simulink model "FMS"  (R2021b)
settings: Solver=VariableStepAuto  StartTime=0.0  StopTime=10.0  RelTol=1e-3
model workspace (MAT data in the model file):
  Control_State_In = Simulink.Bus
  Control_State_In.Alignment = -1
  Control_State_In.PreserveElementDimensions = 0
  Control_State_In.Elements_internal(1) = Simulink.BusElement
  Control_State_In.Elements_internal(1).DimensionsMode = 'Fixed'
  Control_State_In.Elements_internal(1).SamplingMode = 'Sample based'
  Control_State_In.Elements_internal(1).SampleTime = -1
  Control_State_In.Elements_internal(1).Description = 'position'
  Control_State_In.Elements_internal(1).Name = 'x'
  Control_State_In.Elements_internal(1).DataType_internal = 'double'
  Control_State_In.Elements_internal(1).Complexity = 'real'
  Control_State_In.Elements_internal(1).Dimensions = 1
  Control_State_In.Elements_internal(2) = Simulink.BusElement
  Control_State_In.Elements_internal(2).DimensionsMode = 'Fixed'
  Control_State_In.Elements_internal(2).SamplingMode = 'Sample based'
  Control_State_In.Elements_internal(2).SampleTime = -1
  Control_State_In.Elements_internal(2).Description = 'position'
  Control_State_In.Elements_internal(2).Name = 'y'
  Control_State_In.Elements_internal(2).DataType_internal = 'double'
  Control_State_In.Elements_internal(2).Complexity = 'real'
  Control_State_In.Elements_internal(2).Dimensions = 1
  Control_State_In.Elements_internal(3) = Simulink.BusElement
  Control_State_In.Elements_internal(3).DimensionsMode = 'Fixed'
  Control_State_In.Elements_internal(3).SamplingMode = 'Sample based'
  Control_State_In.Elements_internal(3).SampleTime = -1
  Control_State_In.Elements_internal(3).Description = 'cap'
  Control_State_In.Elements_internal(3).Name = 'fpa'
  Control_State_In.Elements_internal(3).DataType_internal = 'double'
  Control_State_In.Elements_internal(3).Complexity = 'real'
  Control_State_In.Elements_internal(3).Dimensions = 1
  Control_State_In.Elements_internal(4) = Simulink.BusElement
  Control_State_In.Elements_internal(4).DimensionsMode = 'Fixed'
  Control_State_In.Elements_internal(4).SamplingMode = 'Sample based'
  Control_State_In.Elements_internal(4).SampleTime = -1
  Control_State_In.Elements_internal(4).Description = 'altitude'
  Control_State_In.Elements_internal(4).Name = 'z'
  Control_State_In.Elements_internal(4).DataType_internal = 'double'
  Control_State_In.Elements_internal(4).Complexity = 'real'
  Control_State_In.Elements_internal(4).Dimensions = 1
  Control_State_In.Elements_internal(5) = Simulink.BusElement
  Control_State_In.Elements_internal(5).DimensionsMode = 'Fixed'
  Control_State_In.Elements_internal(5).SamplingMode = 'Sample based'
  Control_State_In.Elements_internal(5).SampleTime = -1
  Control_State_In.Elements_internal(5).Description = 'vitesse'
  Control_State_In.Elements_internal(5).Name = 'Vp'
  Control_State_In.Elements_internal(5).DataType_internal = 'double'
  Control_State_In.Elements_internal(5).Complexity = 'real'
  Control_State_In.Elements_internal(5).Dimensions = 1
  Control_State_In.Elements_internal(6) = Simulink.BusElement
  Control_State_In.Elements_internal(6).DimensionsMode = 'Fixed'
  Control_State_In.Elements_internal(6).SamplingMode = 'Sample based'
  Control_State_In.Elements_internal(6).SampleTime = -1
  Control_State_In.Elements_internal(6).Description = 'roulis'
  Control_State_In.Elements_internal(6).Name = 'phi'
  Control_State_In.Elements_internal(6).DataType_internal = 'double'
  Control_State_In.Elements_internal(6).Complexity = 'real'
  Control_State_In.Elements_internal(6).Dimensions = 1
  Control_State_In.Elements_internal(7) = Simulink.BusElement
  Control_State_In.Elements_internal(7).DimensionsMode = 'Fixed'
  Control_State_In.Elements_internal(7).SamplingMode = 'Sample based'
  Control_State_In.Elements_internal(7).SampleTime = -1
  Control_State_In.Elements_internal(7).Description = 'lacet'
  Control_State_In.Elements_internal(7).Name = 'psi'
  Control_State_In.Elements_internal(7).DataType_internal = 'double'
  Control_State_In.Elements_internal(7).Complexity = 'real'
  Control_State_In.Elements_internal(7).Dimensions = 1
  Control_State_In.DataScope = 'Auto'
  Pilot_Input = Simulink.Bus
  Pilot_Input.Alignment = -1
  Pilot_Input.PreserveElementDimensions = 0
  Pilot_Input.Elements_internal = Simulink.BusElement
  Pilot_Input.Elements_internal.DimensionsMode = 'Fixed'
  Pilot_Input.Elements_internal.SamplingMode = 'Sample based'
  Pilot_Input.Elements_internal.SampleTime = -1
  Pilot_Input.Elements_internal.Description = 'choix de mode FCU par le pilote'
  Pilot_Input.Elements_internal.Name = 'FCU_lateral_mode'
  Pilot_Input.Elements_internal.DataType_internal = 'int8'
  Pilot_Input.Elements_internal.Complexity = 'real'
  Pilot_Input.Elements_internal.Dimensions = 1
  Pilot_Input.DataScope = 'Auto'
settings Model: Creator=lhubl  LastModifiedBy=Paul

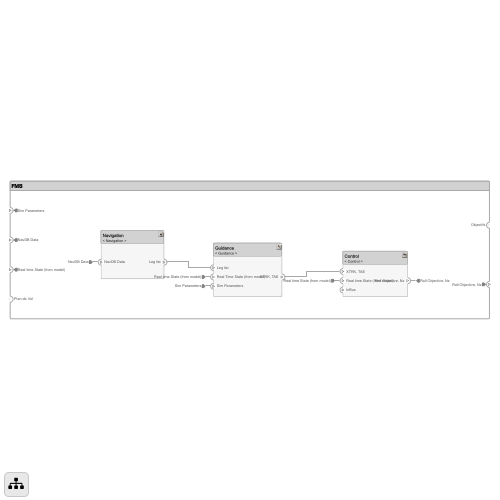
[thumbnail: Simulink's stored preview of the top-level diagram]
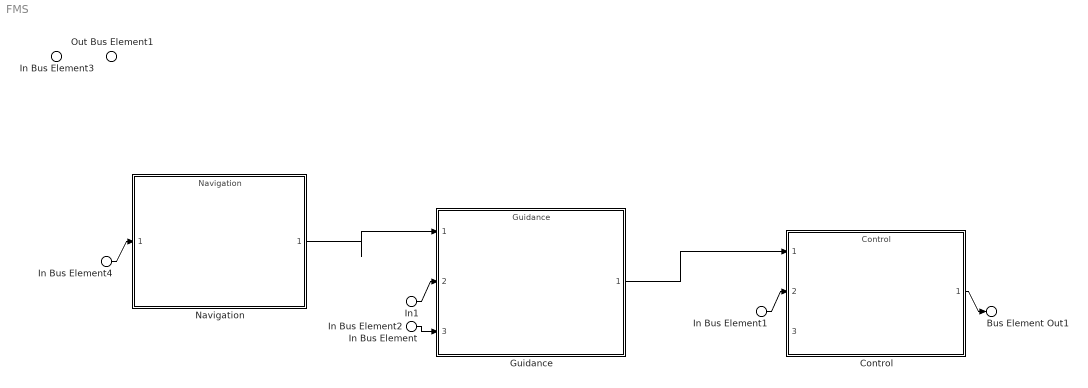
== system FMS ==
  In Bus Element : Inport  PortName=Sim Parameters
  In Bus Element4 : Inport  Port=2  PortName=NavDB Data
  In Bus Element1 : Inport  Port=3  PortName=Real time State (from model)
  In Bus Element2 : Inport  Port=3  PortName=Real time State (from model)
  In1 : Inport  Port=3  PortName=Real time State (from model)
  In Bus Element3 : Inport  Port=4  PortName=Plan de Vol
  Control : ModelReference  ModelNameDialog=Control  SimulationMode=Normal  ModelReferenceVersion=1.4
      settings: PortSchema="{\"entries\":[{\"content\":{\"headerSize\":38,\"margin\":15,\"minimumSpacing\":25,\"sides\":[{\"content\":{\"connectorIds\":[\"In1\",\"In2\",\"In3\"]},\"type\":\"ConnectorPlacement.EquallySpacedRectSide\",\"uuid\":\"f0697a98-65c4-48b6-9148-6d90a1a908b8\"},{\"content\":{\"connectorIds\":[\"Out1\"],\"side\":\"RIGHT\"},\"type\":\"ConnectorPlacement.EquallySpacedRectSide\",\"uuid\":\"c62a382e-4014-433d-b035-2a8a1906ece2\"},{\"content\":{\"connectorIds\":[],\"side\":\"TOP\"},\"type\":\"ConnectorPlacement.EquallySpacedRectSide\",\"uuid\":\"02cc979b-05b8-4cbd-9662-94fbd431603b\"}]},\"type\":\"ConnectorPlacement.EquallySpacedConnector\",\"uuid\":\"1201885f-d543-4e5c-981e-efbc8a5dca28\"}],\"packageUris\":[\"http://schema.mathworks.com/mf0/Connector/R2020b\"],\"version\":\"1.0\"}"
  "Guidance " : ModelReference  ModelNameDialog=Guidance  SimulationMode=Normal  ModelReferenceVersion=1.11
      settings: PortSchema="{\"entries\":[{\"content\":{\"headerSize\":38,\"margin\":15,\"minimumSpacing\":25,\"sides\":[{\"content\":{\"connectorIds\":[\"In1\",\"In2\",\"In3\"]},\"type\":\"ConnectorPlacement.EquallySpacedRectSide\",\"uuid\":\"f0697a98-65c4-48b6-9148-6d90a1a908b8\"},{\"content\":{\"connectorIds\":[\"Out1\"],\"side\":\"RIGHT\"},\"type\":\"ConnectorPlacement.EquallySpacedRectSide\",\"uuid\":\"c62a382e-4014-433d-b035-2a8a1906ece2\"},{\"content\":{\"connectorIds\":[],\"side\":\"TOP\"},\"type\":\"ConnectorPlacement.EquallySpacedRectSide\",\"uuid\":\"02cc979b-05b8-4cbd-9662-94fbd431603b\"}]},\"type\":\"ConnectorPlacement.EquallySpacedConnector\",\"uuid\":\"1201885f-d543-4e5c-981e-efbc8a5dca28\"}],\"packageUris\":[\"http://schema.mathworks.com/mf0/Connector/R2020b\"],\"version\":\"1.0\"}"
  Navigation : ModelReference  ModelNameDialog=Navigation  SimulationMode=Normal  ModelReferenceVersion=1.3
      settings: PortSchema="{\"entries\":[{\"content\":{\"headerSize\":38,\"margin\":15,\"minimumSpacing\":25,\"sides\":[{\"content\":{\"connectorIds\":[\"In1\"]},\"type\":\"ConnectorPlacement.EquallySpacedRectSide\",\"uuid\":\"f0697a98-65c4-48b6-9148-6d90a1a908b8\"},{\"content\":{\"connectorIds\":[\"Out1\"],\"side\":\"RIGHT\"},\"type\":\"ConnectorPlacement.EquallySpacedRectSide\",\"uuid\":\"c62a382e-4014-433d-b035-2a8a1906ece2\"},{\"content\":{\"connectorIds\":[],\"side\":\"TOP\"},\"type\":\"ConnectorPlacement.EquallySpacedRectSide\",\"uuid\":\"02cc979b-05b8-4cbd-9662-94fbd431603b\"}]},\"type\":\"ConnectorPlacement.EquallySpacedConnector\",\"uuid\":\"1201885f-d543-4e5c-981e-efbc8a5dca28\"}],\"packageUris\":[\"http://schema.mathworks.com/mf0/Connector/R2020b\"],\"version\":\"1.0\"}"
  Out Bus Element1 : Outport  PortName=Objectifs
  Bus Element Out1 : Outport  RequirementInfo={} %GIDa_68c6b491_cecf_42b1_babe_de608741fe37  Port=2  PortName=Roll Objective, Nz
  wires:
  Navigation/1 -> "Guidance "/1
  In Bus Element1/1 -> Control/2
  "Guidance "/1 -> Control/1
  Control/1 -> Bus Element Out1/1
  In Bus Element4/1 -> Navigation/1
  In Bus Element/1 -> "Guidance "/3
  In1/1 -> "Guidance "/2
